simulink model "es2_rif"  (R2014a)
settings: Solver=ode45  StartTime=0.0  StopTime=20.0  RelTol=1e-3
values from neighbouring files (symbols this model uses):
  Kr = 2    [es2.m]
libraries: cstblocks x2, simulink x1
settings Model: Creator=HP  LastModifiedBy=HP

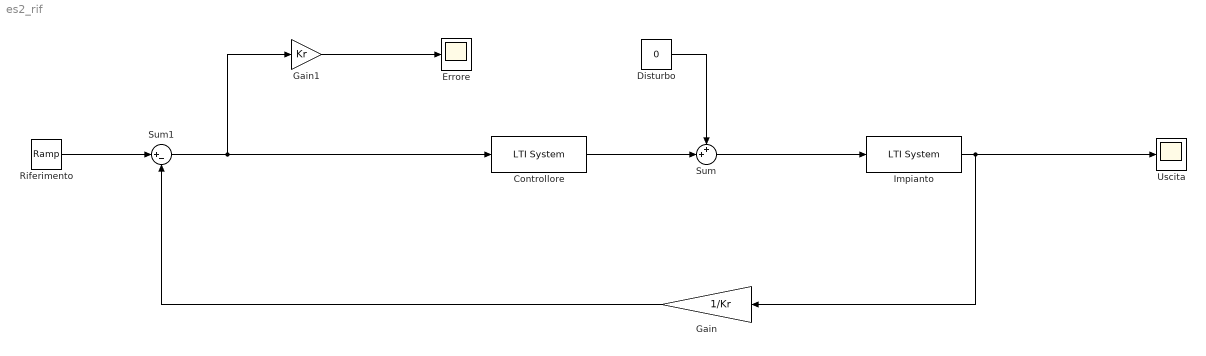
== system es2_rif ==
  Controllore : cstblocks/LTI System  sys=C  IC=[]
  Disturbo : Constant  Value=0
  Errore : Scope
  Gain : Gain  Gain=1/Kr
  Gain1 : Gain  Gain=Kr
  Impianto : cstblocks/LTI System  sys=F  IC=[]
  Riferimento : simulink/Sources/Ramp  slope=1  start=0  X0=0
  Sum : Sum  Inputs=++|
  Sum1 : Sum  Inputs=|+-
  Uscita : Scope
  wires:
  Controllore/1 -> Sum/2
  Sum/1 -> Impianto/1
  Sum1/1 -> Gain1/1, Controllore/1
  Gain/1 -> Sum1/2
  Riferimento/1 -> Sum1/1
  Disturbo/1 -> Sum/1
  Impianto/1 -> Uscita/1, Gain/1
  Gain1/1 -> Errore/1
